simulink model "packetizer_core"  (R2016b)
settings: Solver=VariableStepAuto  StartTime=0.0  StopTime=2*64*512+100  RelTol=1e-3
model workspace (MAT data in the model file):
  dstin = [0 168430081 168430082 168430083 168430084 168430085 168430086 168430087 168430088 168430089 168430090 168430091 168430092 168430093 168430094 168430095 168430096 168430097 168430098 168430099 168430100 168430101 168430102 168430103 168430104 168430105 168430106 168430107 168430108 168430109 168430110 168430111 168430112]
  simin = [1 2 3 4 5 6 7 8 9 10 11 12 ... (262544 elements, 65636x4)]
libraries: xbsIndex_r4 x142
(part 1 of 2)
settings Model: Creator=davidm  LastModifiedBy=davidm

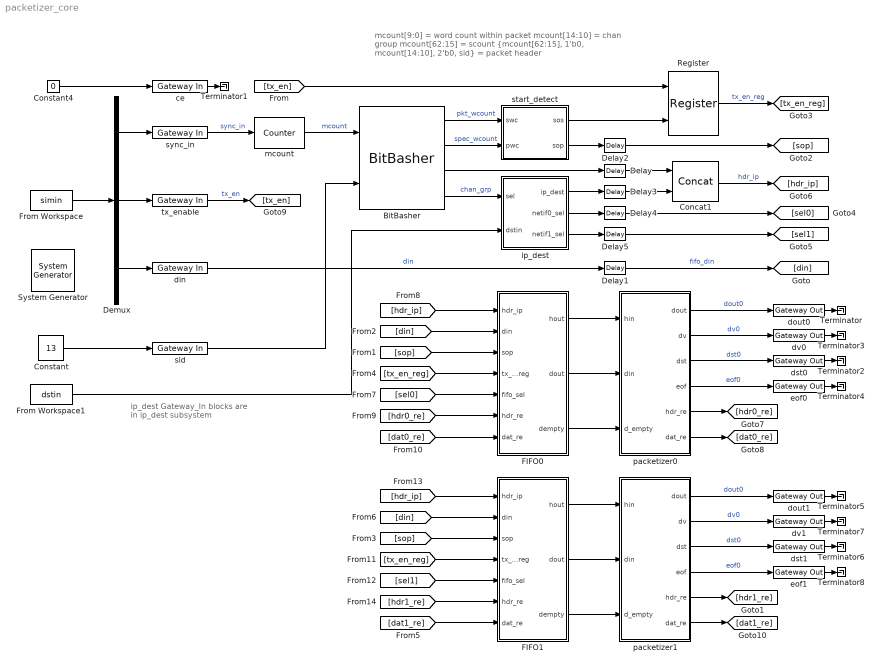
== system packetizer_core ==
  note: ip_dest Gateway_In blocks
      | are in ip_dest subsystem
  note: mcount[9:0] = word count within packet
      | mcount[14:10] = chan group
      | mcount[62:15] = scount
      | {mcount[62:15], 1'b0, mcount[14:10], 2'b0, sid} = packet header
  " System Generator" : xbsIndex_r4/ System Generator  Tag=genX  xilinxfamily=kintex7  part=xc7k160t  speed=-2  package=ffg676  synthesis_tool=XST  clock_wrapper=Clock Enables  directory=./packetizer_core  proj_type=Project Navigator  Synth_file=XST Defaults  Impl_file=ISE Defaults  testbench=off  simulink_period=1  sysclk_period=10  dcm_input_clock_period=10  incr_netlist=off  trim_vbits=Everywhere in SubSystem  dbl_ovrd=According to Block Masks  core_generation=According to Block Masks  run_coregen=off  deprecated_control=off  eval_field=0  block_type=sysgen
  BitBasher : xbsIndex_r4/BitBasher  bitexpr=|  display_expr=off  sr_1=spec_wcount  arith_type1=Unsigned  bin_pt1=0  sr_2=pkt_wcount  arith_type2=Unsigned  bin_pt2=0  sr_3=header  arith_type3=Unsigned  bin_pt3=0  sr_4=chan_grp  arith_type4=Unsigned  bin_pt4=0  dbl_ovrd=off  block_type=bitbasher
      | spec_wcount={mcount[14:0]}
      | pkt_wcount={mcount[9:0]}
      | header={mcount[62:15], 1'b0, mcount[14:10], 2'b0, sid}
      | chan_grp={mcount[14:10]}
  Concat1 : xbsIndex_r4/Concat  num_inputs=2  dbl_ovrd=off  block_type=concat
  Constant : Constant  Value=13
  Constant4 : Constant  Value=0
  Delay : xbsIndex_r4/Delay  rst=off  infoeditControl=Selection of Reset will increase slice count due to use of real FFs and instead of SRLs  en=off  latency=2  reg_retiming=off  dbl_ovrd=off  block_type=delay
  Delay1 : xbsIndex_r4/Delay  rst=off  infoeditControl=Selection of Reset will increase slice count due to use of real FFs and instead of SRLs  en=off  latency=2  reg_retiming=off  dbl_ovrd=off  block_type=delay
  Delay{2..5} (4 alike) : xbsIndex_r4/Delay  rst=off  infoeditControl=Selection of Reset will increase slice count due to use of real FFs and instead of SRLs  en=off  latency=1  reg_retiming=off  dbl_ovrd=off  block_type=delay
  Demux : Demux  Outputs=3
  FIFO0 : Subsystem
  FIFO1 : Subsystem
  From Workspace : FromWorkspace  VariableName=simin  SampleTime=0  OutputAfterFinalValue=Holding final value
  From Workspace1 : FromWorkspace  VariableName=dstin  SampleTime=0  Interpolate=off  OutputAfterFinalValue=Holding final value
  Register : xbsIndex_r4/Register  init=0  rst=off  en=on  dbl_ovrd=off  block_type=register
  Terminator{,1..8} (9 alike) : Terminator
  ce : xbsIndex_r4/Gateway In  gui_display_data_type=Fixed-point  arith_type=Unsigned  n_bits=1  bin_pt=0  preci_type=Single  exp_width=8  frac_width=24  rows=1  columns=1  quantization="Round  (unbiased: +/- Inf)"  overflow=Saturate  period=1  UseAsADC=off  ADCChannel='1'  interface=None  automatic_assignment=on  address_offset=hex2dec('00')  intf_name=''  intf_description=''  default_value=0  timing_constraint=None  locs_specified=off  LOCs={}  io_standard={}  inherit_from_input=off  hdl_port=on  dbl_ovrd=off  block_type=gatewayin
  din : xbsIndex_r4/Gateway In  gui_display_data_type=Fixed-point  arith_type=Unsigned  n_bits=64  bin_pt=0  preci_type=Single  exp_width=8  frac_width=24  rows=1  columns=1  quantization="Round  (unbiased: +/- Inf)"  overflow=Saturate  period=1  UseAsADC=off  ADCChannel='1'  interface=None  automatic_assignment=on  address_offset=hex2dec('00')  intf_name=''  intf_description=''  default_value=0  timing_constraint=None  locs_specified=off  LOCs={}  io_standard={}  inherit_from_input=off  hdl_port=on  dbl_ovrd=off  block_type=gatewayin
  dout0 : xbsIndex_r4/Gateway Out  inherit_from_input=off  hdl_port=on  rows=1  columns=1  UseAsDAC=off  DACChannel='1'  interface=None  automatic_assignment=on  address_offset=hex2dec('00')  intf_name=''  intf_description=''  timing_constraint=None  locs_specified=off  LOCs={}  io_standard={}  block_type=gatewayout
  dout1 : xbsIndex_r4/Gateway Out  inherit_from_input=off  hdl_port=on  rows=1  columns=1  UseAsDAC=off  DACChannel='1'  interface=None  automatic_assignment=on  address_offset=hex2dec('00')  intf_name=''  intf_description=''  timing_constraint=None  locs_specified=off  LOCs={}  io_standard={}  block_type=gatewayout
  dst0 : xbsIndex_r4/Gateway Out  inherit_from_input=off  hdl_port=on  rows=1  columns=1  UseAsDAC=off  DACChannel='1'  interface=None  automatic_assignment=on  address_offset=hex2dec('00')  intf_name=''  intf_description=''  timing_constraint=None  locs_specified=off  LOCs={}  io_standard={}  block_type=gatewayout
  dst1 : xbsIndex_r4/Gateway Out  inherit_from_input=off  hdl_port=on  rows=1  columns=1  UseAsDAC=off  DACChannel='1'  interface=None  automatic_assignment=on  address_offset=hex2dec('00')  intf_name=''  intf_description=''  timing_constraint=None  locs_specified=off  LOCs={}  io_standard={}  block_type=gatewayout
  dv0 : xbsIndex_r4/Gateway Out  inherit_from_input=off  hdl_port=on  rows=1  columns=1  UseAsDAC=off  DACChannel='1'  interface=None  automatic_assignment=on  address_offset=hex2dec('00')  intf_name=''  intf_description=''  timing_constraint=None  locs_specified=off  LOCs={}  io_standard={}  block_type=gatewayout
  dv1 : xbsIndex_r4/Gateway Out  inherit_from_input=off  hdl_port=on  rows=1  columns=1  UseAsDAC=off  DACChannel='1'  interface=None  automatic_assignment=on  address_offset=hex2dec('00')  intf_name=''  intf_description=''  timing_constraint=None  locs_specified=off  LOCs={}  io_standard={}  block_type=gatewayout
  eof0 : xbsIndex_r4/Gateway Out  inherit_from_input=off  hdl_port=on  rows=1  columns=1  UseAsDAC=off  DACChannel='1'  interface=None  automatic_assignment=on  address_offset=hex2dec('00')  intf_name=''  intf_description=''  timing_constraint=None  locs_specified=off  LOCs={}  io_standard={}  block_type=gatewayout
  eof1 : xbsIndex_r4/Gateway Out  inherit_from_input=off  hdl_port=on  rows=1  columns=1  UseAsDAC=off  DACChannel='1'  interface=None  automatic_assignment=on  address_offset=hex2dec('00')  intf_name=''  intf_description=''  timing_constraint=None  locs_specified=off  LOCs={}  io_standard={}  block_type=gatewayout
  ip_dest : Subsystem
  mcount : xbsIndex_r4/Counter  cnt_type=Free Running  cnt_to=Inf  operation=Up  start_count=0  cnt_by_val=1  arith_type=Unsigned  n_bits=48+6+5+10  bin_pt=0  load_pin=off  rst=on  en=off  explicit_period=on  period=1  use_behavioral_HDL=off  implementation=Fabric  dbl_ovrd=off  block_type=counter
  packetizer0 : Subsystem
  packetizer1 : Subsystem
  sid : xbsIndex_r4/Gateway In  gui_display_data_type=Fixed-point  arith_type=Unsigned  n_bits=8  bin_pt=0  preci_type=Single  exp_width=8  frac_width=24  rows=1  columns=1  quantization="Round  (unbiased: +/- Inf)"  overflow=Saturate  period=1  UseAsADC=off  ADCChannel='1'  interface=None  automatic_assignment=on  address_offset=hex2dec('00')  intf_name=''  intf_description=''  default_value=0  timing_constraint=None  locs_specified=off  LOCs={}  io_standard={}  inherit_from_input=off  hdl_port=on  dbl_ovrd=off  block_type=gatewayin
  start_detect : Subsystem
  sync_in : xbsIndex_r4/Gateway In  gui_display_data_type=Boolean  arith_type=Boolean  n_bits=16  bin_pt=14  preci_type=Single  exp_width=8  frac_width=24  rows=1  columns=1  quantization="Round  (unbiased: +/- Inf)"  overflow=Saturate  period=1  UseAsADC=off  ADCChannel='1'  interface=None  automatic_assignment=on  address_offset=hex2dec('00')  intf_name=''  intf_description=''  default_value=0  timing_constraint=None  locs_specified=off  LOCs={}  io_standard={}  inherit_from_input=off  hdl_port=on  dbl_ovrd=off  block_type=gatewayin
  tx_enable : xbsIndex_r4/Gateway In  gui_display_data_type=Boolean  arith_type=Boolean  n_bits=64  bin_pt=0  preci_type=Single  exp_width=8  frac_width=24  rows=1  columns=1  quantization="Round  (unbiased: +/- Inf)"  overflow=Saturate  period=1  UseAsADC=off  ADCChannel='1'  interface=None  automatic_assignment=on  address_offset=hex2dec('00')  intf_name=''  intf_description=''  default_value=0  timing_constraint=None  locs_specified=off  LOCs={}  io_standard={}  inherit_from_input=off  hdl_port=on  dbl_ovrd=off  block_type=gatewayin
  wires:
  From Workspace/1 -> Demux/1
  Demux/1 -> sync_in/1
  Constant4/1 -> ce/1
  ce/1 -> Terminator1/1
  From Workspace1/1 -> ip_dest/2(dstin)
  Constant/1 -> sid/1
  mcount/1 -> BitBasher/1  "mcount"
  sid/1 -> BitBasher/2
  BitBasher/4 -> ip_dest/1(sel)  "chan_grp"
  sync_in/1 -> mcount/1  "sync_in"
  BitBasher/1 -> start_detect/1(swc)  "pkt_wcount"
  BitBasher/2 -> start_detect/2(pwc)  "spec_wcount"
  din/1 -> Delay1/1  "din"
  tx_enable/1 -> [tx_en]  "tx_en"
  [tx_en] -> Register/1
  Register/1 -> [tx_en_reg]  "tx_en_reg"
  ip_dest/2(netif0_sel) -> Delay4/1
  ip_dest/3(netif1_sel) -> Delay5/1
  BitBasher/3 -> Delay/1
  ip_dest/1(ip_dest) -> Delay3/1
  Concat1/1 -> [hdr_ip]  "hdr_ip"
  start_detect/2(sop) -> Delay2/1
  Demux/2 -> tx_enable/1
  Demux/3 -> din/1
  Delay/1 -> Concat1/1
  start_detect/1(sos) -> Register/2
  Delay2/1 -> [sop]
  Delay3/1 -> Concat1/2
  Delay4/1 -> [sel0]
  Delay5/1 -> [sel1]
  Delay1/1 -> [din]  "fifo_din"
  [hdr_ip] -> FIFO0/1(hdr_ip)
  [din] -> FIFO0/2(din)
  [sop] -> FIFO0/3(sop)
  [tx_en_reg] -> FIFO0/4(tx_en_reg)
  [sel0] -> FIFO0/5(fifo_sel)
  [hdr0_re] -> FIFO0/6(hdr_re)
  [dat0_re] -> FIFO0/7(dat_re)
  FIFO0/1(hout) -> packetizer0/1(hin)
  FIFO0/2(dout) -> packetizer0/2(din)
  FIFO0/3(dempty) -> packetizer0/3(d_empty)
  packetizer0/5(hdr_re) -> [hdr0_re]
  packetizer0/6(dat_re) -> [dat0_re]
  packetizer0/1(dout) -> dout0/1  "dout0"
  packetizer0/2(dv) -> dv0/1  "dv0"
  packetizer0/3(dst) -> dst0/1  "dst0"
  packetizer0/4(eof) -> eof0/1  "eof0"
  dout0/1 -> Terminator/1
  dst0/1 -> Terminator2/1
  dv0/1 -> Terminator3/1
  eof0/1 -> Terminator4/1
  [hdr_ip] -> FIFO1/1(hdr_ip)
  [din] -> FIFO1/2(din)
  [sop] -> FIFO1/3(sop)
  [tx_en_reg] -> FIFO1/4(tx_en_reg)
  [sel1] -> FIFO1/5(fifo_sel)
  [hdr1_re] -> FIFO1/6(hdr_re)
  [dat1_re] -> FIFO1/7(dat_re)
  FIFO1/1(hout) -> packetizer1/1(hin)
  FIFO1/2(dout) -> packetizer1/2(din)
  FIFO1/3(dempty) -> packetizer1/3(d_empty)
  packetizer1/5(hdr_re) -> [hdr1_re]
  packetizer1/6(dat_re) -> [dat1_re]
  packetizer1/1(dout) -> dout1/1  "dout0"
  packetizer1/2(dv) -> dv1/1  "dv0"
  packetizer1/3(dst) -> dst1/1  "dst0"
  packetizer1/4(eof) -> eof1/1  "eof0"
  dout1/1 -> Terminator5/1
  dst1/1 -> Terminator6/1
  dv1/1 -> Terminator7/1
  eof1/1 -> Terminator8/1
